simulink model "DCmotorSimulink_speed_control_motor"  (R2023b)
settings: Solver=VariableStepAuto  StartTime=0.0  StopTime=10  RelTol=1e-3
values from neighbouring files (symbols this model uses):
  J = 0.068    [DCmotor_speed_control_parameter.m]
  Ka = 1    [DCmotor_speed_control_parameter.m]
  La = 2.3e-3    (= 0.0023)    [DCmotor_speed_control_parameter.m]
  M = 1.304    [DCmotor_speed_control_parameter.m]
  R_f = 356.7    [DCmotor_speed_control_parameter.m]
  Ra = 0.3    [DCmotor_speed_control_parameter.m]
  speed_ref = 20    [DCmotor_speed_control_parameter.m]
  Tload = 0    [DCmotor_speed_control_parameter.m]
undefined symbols (not defined in the file or in its folder): Pmax, v_f_rated, v_t_rated
libraries: slpidlib x2
settings Model: Creator=chayutht  LastModifiedBy=chayutht

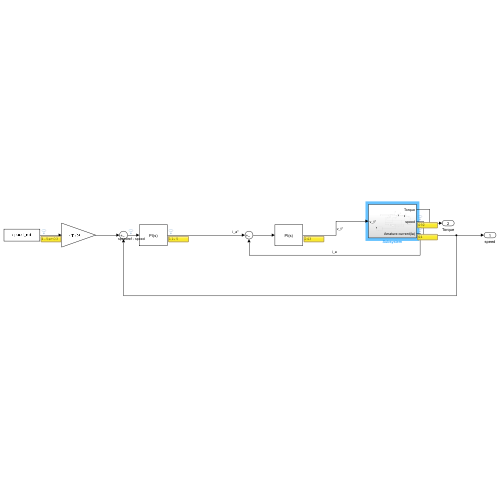
[thumbnail: Simulink's stored preview of the top-level diagram]
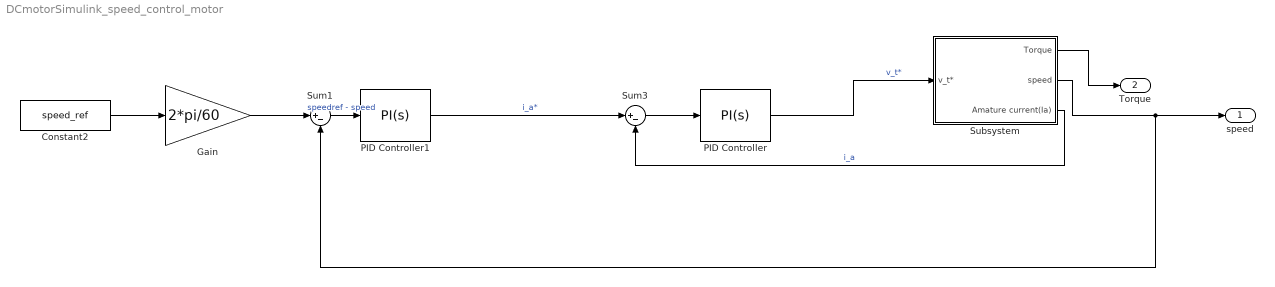
== system DCmotorSimulink_speed_control_motor ==
  Constant2 : Constant  Value=speed_ref
  Gain : Gain  Gain=2*pi/60
  PID Controller : slpidlib/PID Controller  Controller=PI  Form=Parallel  TimeDomain=Continuous-time  UseExternalTs=off  SampleTime=-1  IntegratorMethod=Forward Euler  FilterMethod=Forward Euler  ControllerParametersSource=internal  P=1  I=1  UseKiTs=off  D=0  N=100  UseFilter=on  TunerSelectOption=Transfer Function Based (PID Tuner App)  InitialConditionSource=internal  InitialConditionForIntegrator=0  InitialConditionForFilter=0  DifferentiatorICPrevScaledInput=0  ExternalReset=none  TrackingMode=off  Kt=1  LimitOutput=off  SatLimitsSource=internal  UpperSaturationLimit=inf  LowerSaturationLimit=-inf  LinearizeAsGain=on  AntiWindupMode=none  Kb=1  LimitIntegrator=off  UpperIntegratorSaturationLimit=inf  LowerIntegratorSaturationLimit=-inf  POutMin=[]  POutMax=[]  IOutMin=[]  IOutMax=[]  DOutMin=[]  DOutMax=[]  NOutMin=[]  NOutMax=[]  SumOutMin=[]  SumOutMax=[]  SaturationOutMin=[]  SaturationOutMax=[]  PParamMin=[]  PParamMax=[]  IParamMin=[]  IParamMax=[]  DParamMin=[]  DParamMax=[]  NParamMin=[]  NParamMax=[]  KbParamMin=[]  KbParamMax=[]  KtParamMin=[]  KtParamMax=[]  KbOutMin=[]  KbOutMax=[]  KtOutMin=[]  KtOutMax=[]  IntegratorOutMin=[]  IntegratorOutMax=[]  FilterOutMin=[]  FilterOutMax=[]  SumI1OutMin=[]  SumI1OutMax=[]  SumI2OutMin=[]  SumI2OutMax=[]  SumI3OutMin=[]  SumI3OutMax=[]  SumI4OutMin=[]  SumI4OutMax=[]  SumDOutMin=[]  SumDOutMax=[]  DifferentiatorOutMin=[]  DifferentiatorOutMax=[]  FilterDiffOutCoefMin=[]  FilterDiffOutCoefMax=[]  ReciprocalOutMin=[]  ReciprocalOutMax=[]  SumDenOutMin=[]  SumDenOutMax=[]  SumNumOutMin=[]  SumNumOutMax=[]  DivideOutMin=[]  DivideOutMax=[]  UdiffTsProdOutMin=[]  UdiffTsProdOutMax=[]  NTsProdOutMin=[]  NTsProdOutMax=[]  UintegralTsProdOutMin=[]  UintegralTsProdOutMax=[]  UngainTsProdOutMin=[]  UngainTsProdOutMax=[]  ClampingZeroOutDataTypeStr=Inherit: Inherit via back propagation  ClampingZeroOutMin=[]  ClampingZeroOutMax=[]  FilterDenConstantOutDataTypeStr=Inherit: Inherit via back propagation  FilterDenConstantOutMin=[]  FilterDenConstantOutMax=[]  PCopyOutDataTypeStr=Inherit: Inherit via back propagation  PCopyOutMin=[]  PCopyOutMax=[]  NCopyOutDataTypeStr=Inherit: Inherit via back propagation  NCopyOutMin=[]  NCopyOutMax=[]  IntegratorContinuousStateAttributes=''  IntegratorStateMustResolveToSignalObject=off  IntegratorRTWStateStorageClass=Auto  FilterContinuousStateAttributes=''  FilterStateMustResolveToSignalObject=off  FilterRTWStateStorageClass=Auto  ParallelPVariant=InternalParameters  IdealPVariant=Disabled  IVariant=InternalParameters  DVariant=Disabled  IntegratorVariant=Continuous  SatVariant=Disabled  AWVariant=Passthrough  PCopyVariant=Disabled  TRVariant=Disabled  FdbkBlocksVariant=Forward  IdealPFdbkVariant=Disabled  SatFdbkVariant=Disabled  DerivativeFilterVariant=Disabled  NVariant=Disabled  NCopyVariant=Disabled_SignalSpec  FilterICVariant=Disabled  IntegratorICVariant=InternalICs  ExternalResetVariant=Disabled  TRSumVariant=Passthrough  SumFdbkVariant=Disabled  SumVariant=Sum_PI  TsampFilterVariant=InternalTs  TsampNgainVariant=Passthrough  TsampIntegralVariant=Disabled_SignalSpec  ExternalSaturationOutDataTypeStr=Inherit: Same as second input
  PID Controller1 : slpidlib/PID Controller  Controller=PI  Form=Parallel  TimeDomain=Continuous-time  UseExternalTs=off  SampleTime=-1  IntegratorMethod=Forward Euler  FilterMethod=Forward Euler  ControllerParametersSource=internal  P=0.5  I=1  UseKiTs=off  D=0  N=100  UseFilter=on  TunerSelectOption=Transfer Function Based (PID Tuner App)  InitialConditionSource=internal  InitialConditionForIntegrator=0  InitialConditionForFilter=0  DifferentiatorICPrevScaledInput=0  ExternalReset=none  TrackingMode=off  Kt=1  LimitOutput=off  SatLimitsSource=internal  UpperSaturationLimit=inf  LowerSaturationLimit=-inf  LinearizeAsGain=on  AntiWindupMode=none  Kb=1  LimitIntegrator=off  UpperIntegratorSaturationLimit=inf  LowerIntegratorSaturationLimit=-inf  POutMin=[]  POutMax=[]  IOutMin=[]  IOutMax=[]  DOutMin=[]  DOutMax=[]  NOutMin=[]  NOutMax=[]  SumOutMin=[]  SumOutMax=[]  SaturationOutMin=[]  SaturationOutMax=[]  PParamMin=[]  PParamMax=[]  IParamMin=[]  IParamMax=[]  DParamMin=[]  DParamMax=[]  NParamMin=[]  NParamMax=[]  KbParamMin=[]  KbParamMax=[]  KtParamMin=[]  KtParamMax=[]  KbOutMin=[]  KbOutMax=[]  KtOutMin=[]  KtOutMax=[]  IntegratorOutMin=[]  IntegratorOutMax=[]  FilterOutMin=[]  FilterOutMax=[]  SumI1OutMin=[]  SumI1OutMax=[]  SumI2OutMin=[]  SumI2OutMax=[]  SumI3OutMin=[]  SumI3OutMax=[]  SumI4OutMin=[]  SumI4OutMax=[]  SumDOutMin=[]  SumDOutMax=[]  DifferentiatorOutMin=[]  DifferentiatorOutMax=[]  FilterDiffOutCoefMin=[]  FilterDiffOutCoefMax=[]  ReciprocalOutMin=[]  ReciprocalOutMax=[]  SumDenOutMin=[]  SumDenOutMax=[]  SumNumOutMin=[]  SumNumOutMax=[]  DivideOutMin=[]  DivideOutMax=[]  UdiffTsProdOutMin=[]  UdiffTsProdOutMax=[]  NTsProdOutMin=[]  NTsProdOutMax=[]  UintegralTsProdOutMin=[]  UintegralTsProdOutMax=[]  UngainTsProdOutMin=[]  UngainTsProdOutMax=[]  ClampingZeroOutDataTypeStr=Inherit: Inherit via back propagation  ClampingZeroOutMin=[]  ClampingZeroOutMax=[]  FilterDenConstantOutDataTypeStr=Inherit: Inherit via back propagation  FilterDenConstantOutMin=[]  FilterDenConstantOutMax=[]  PCopyOutDataTypeStr=Inherit: Inherit via back propagation  PCopyOutMin=[]  PCopyOutMax=[]  NCopyOutDataTypeStr=Inherit: Inherit via back propagation  NCopyOutMin=[]  NCopyOutMax=[]  IntegratorContinuousStateAttributes=''  IntegratorStateMustResolveToSignalObject=off  IntegratorRTWStateStorageClass=Auto  FilterContinuousStateAttributes=''  FilterStateMustResolveToSignalObject=off  FilterRTWStateStorageClass=Auto  ParallelPVariant=InternalParameters  IdealPVariant=Disabled  IVariant=InternalParameters  DVariant=Disabled  IntegratorVariant=Continuous  SatVariant=Disabled  AWVariant=Passthrough  PCopyVariant=Disabled  TRVariant=Disabled  FdbkBlocksVariant=Forward  IdealPFdbkVariant=Disabled  SatFdbkVariant=Disabled  DerivativeFilterVariant=Disabled  NVariant=Disabled  NCopyVariant=Disabled_SignalSpec  FilterICVariant=Disabled  IntegratorICVariant=InternalICs  ExternalResetVariant=Disabled  TRSumVariant=Passthrough  SumFdbkVariant=Disabled  SumVariant=Sum_PI  TsampFilterVariant=InternalTs  TsampNgainVariant=Passthrough  TsampIntegralVariant=Disabled_SignalSpec  ExternalSaturationOutDataTypeStr=Inherit: Same as second input
  Subsystem : Subsystem
  Sum1 : Sum  Inputs=|+-
  Sum3 : Sum  Inputs=|+-
  speed : Outport
  Torque : Outport  Port=2
  wires:
  Sum3/1 -> PID Controller/1
  PID Controller/1 -> Subsystem/1(v_t*)  "v_t*"
  Subsystem/1(Torque) -> Torque/1
  Subsystem/2(speed) -> Sum1/2, speed/1
  Subsystem/3(Amature current(Ia)) -> Sum3/2  "i_a"
  PID Controller1/1 -> Sum3/1  "i_a*"
  Sum1/1 -> PID Controller1/1  "speedref - speed"
  Constant2/1 -> Gain/1
  Gain/1 -> Sum1/1

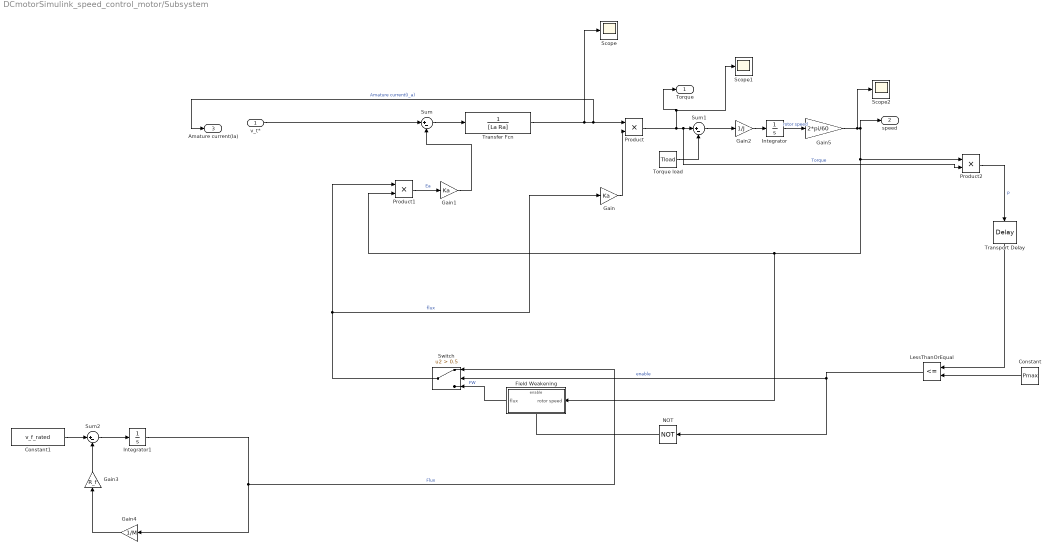
== system DCmotorSimulink_speed_control_motor/Subsystem ==
  v_t* : Inport
  Constant : Constant  Value=Pmax
  Constant1 : Constant  Value=v_f_rated
  Field Weakening : Subsystem  TreatAsAtomicUnit=on
  Gain : Gain  Gain=Ka
  Gain1 : Gain  Gain=Ka
  Gain2 : Gain  Gain=1/J
  Gain3 : Gain  Gain=R_f
  Gain4 : Gain  Gain=1/M
  Gain5 : Gain  Gain=2*pi/60
  Integrator : Integrator  InitialCondition=52.3599
  Integrator1 : Integrator  InitialCondition=0.8476
  LessThanOrEqual : RelationalOperator  Operator=<=  OutDataTypeStr=boolean  RndMeth=Simplest  InputSameDT=off
  NOT : Logic  Operator=NOT  IconShape=distinctive  AllPortsSameDT=off  OutDataTypeStr=boolean
  Product : Product
  Product1 : Product
  Product2 : Product
  Scope : Scope
  Scope1 : Scope
  Scope2 : Scope
  Sum : Sum  Inputs=|+-
  Sum1 : Sum  Inputs=|+-
  Sum2 : Sum  Inputs=|+-
  Switch : Switch  Criteria=u2 > Threshold  Threshold=0.5  SaturateOnIntegerOverflow=off  InputSameDT=off
  Torque load : Constant  Value=Tload
  Transfer Fcn : TransferFcn  Denominator=[La Ra]
      settings: AttributesFormatString=%<Denominator>=(0.5 1)
  Transport Delay : TransportDelay  DelayTime=0.001
  Torque : Outport
  speed : Outport  Port=2
  Amature current(Ia) : Outport  Port=3
  wires:
  Gain/1 -> Product/2
  Integrator/1 -> Gain5/1  "rotor speed"
  Torque load/1 -> Sum1/2
  Integrator1/1 -> Switch/1, Gain4/1  "Flux"
  Sum1/1 -> Gain2/1
  v_t*/1 -> Sum/1
  Product/1 -> Torque/1, Scope1/1, Product2/2, Sum1/1  "Torque"
  Gain2/1 -> Integrator/1
  Gain3/1 -> Sum2/2
  Gain1/1 -> Sum/2
  Product1/1 -> Gain1/1  "Ea"
  Gain4/1 -> Gain3/1
  Transfer Fcn/1 -> Scope/1, Amature current(Ia)/1, Product/1  "Amature current(I_a)"
  Sum2/1 -> Integrator1/1
  Sum/1 -> Transfer Fcn/1
  Constant1/1 -> Sum2/1
  Constant/1 -> LessThanOrEqual/2
  Switch/1 -> Gain/1, Product1/1  "flux"
  LessThanOrEqual/1 -> NOT/1, Switch/2  "enable"
  Product2/1 -> Transport Delay/1  "P"
  Transport Delay/1 -> LessThanOrEqual/1
  Field Weakening/1(flux) -> Switch/3  "FW"
  NOT/1 -> Field Weakening/Enable
  Gain5/1 -> speed/1, Product2/1, Field Weakening/1(rotor speed), Product1/2, Scope2/1

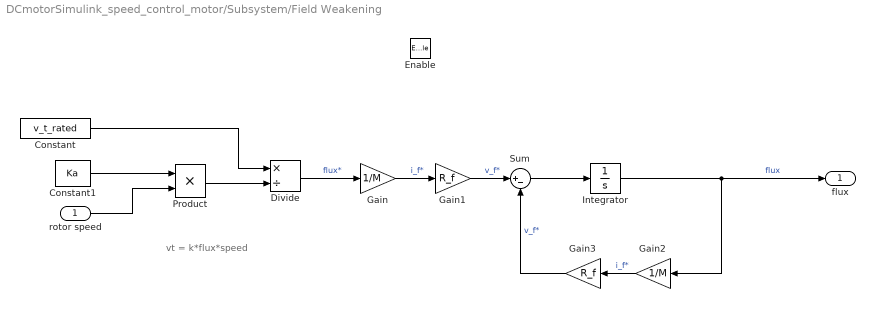
== system DCmotorSimulink_speed_control_motor/Subsystem/Field Weakening ==
  note: vt = k*flux*speed
  rotor speed : Inport
  Enable : EnablePort
  Constant : Constant  Value=v_t_rated
  Constant1 : Constant  Value=Ka
  Divide : Product  Inputs=*/
  Gain : Gain  Gain=1/M
  Gain1 : Gain  Gain=R_f
  Gain2 : Gain  Gain=1/M
  Gain3 : Gain  Gain=R_f
  Integrator : Integrator  InitialCondition=0.848
  Product : Product
  Sum : Sum  Inputs=|+-
  flux : Outport
  wires:
  Constant1/1 -> Product/1
  rotor speed/1 -> Product/2
  Product/1 -> Divide/2
  Constant/1 -> Divide/1
  Divide/1 -> Gain/1  "flux*"
  Gain/1 -> Gain1/1  "i_f*"
  Gain1/1 -> Sum/1  "v_f*"
  Sum/1 -> Integrator/1
  Integrator/1 -> Gain2/1, flux/1  "flux"
  Gain2/1 -> Gain3/1  "i_f*"
  Gain3/1 -> Sum/2  "v_f*"
